simulink model "simulazione_sistema_lineare"  (R2025b)
settings: Solver=VariableStepAuto  StartTime=0.0  StopTime=10.0  RelTol=1e-3
values from neighbouring files (symbols this model uses):
  D_A = 1.5    [simulazione_sistema_non_lineare_code.m]
  D_F = zeros(1,4)    [simulazione_sistema_lineare_code.m]    (also in simulazione_sistema_non_lineare_code.m)
  G = tf(modello)    [tank_in_cascata_costanti.m]
  N_A = 0.1    [simulazione_sistema_non_lineare_code.m]
  N_F = zeros(1,4)    [simulazione_sistema_lineare_code.m]    (also in simulazione_sistema_non_lineare_code.m)
  RR = RR_s*RR_d    [tank_in_cascata_costanti.m]
  W = 3.5    [animazione_regolatore.m]    (also in simulazione_sistema_lineare_code.m = 1; simulazione_sistema_non_lineare_code.m = 1; tank_test_disturbo_dominio_complesso.m; tank_test_disturbo_dominio_tempo.m)
  x0 = [0,0]    [tank_animazione.m]
settings Model: Creator=lucia  LastModifiedBy=ecanf

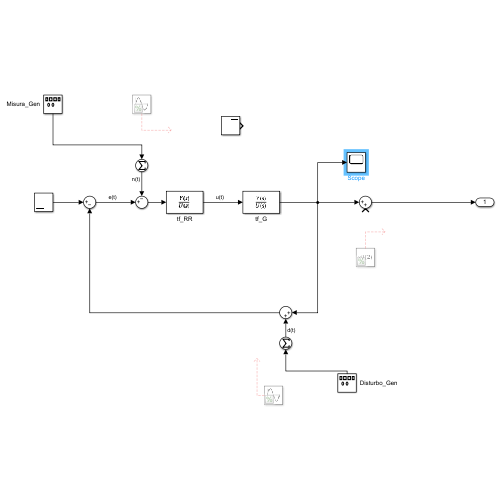
[thumbnail: Simulink's stored preview of the top-level diagram]
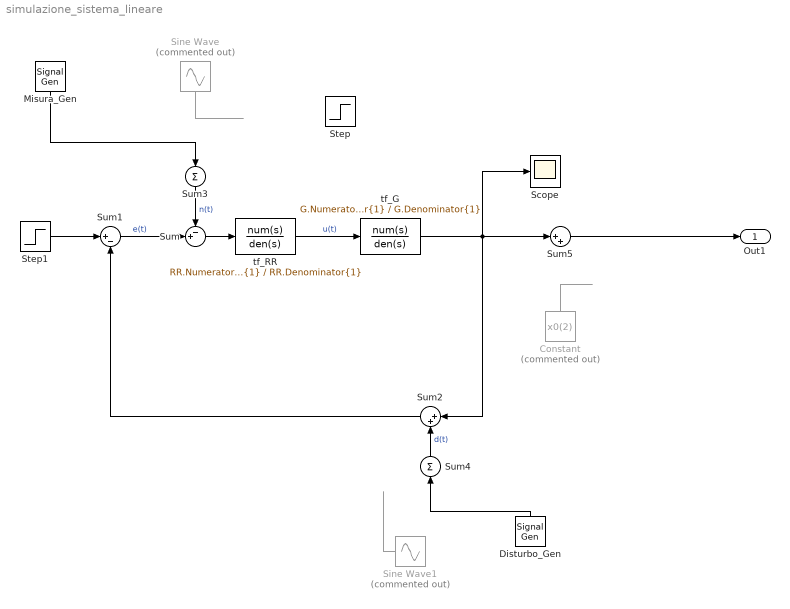
== system simulazione_sistema_lineare ==
  Constant : Constant  Commented=on  Value=x0(2)
  Disturbo_Gen : SignalGenerator  Amplitude="[1.5         1.5         1.5         1.5]"  Frequency="[0.4         0.8         1.2         1.6]"  Units=rad/sec
  Misura_Gen : SignalGenerator  Amplitude="[0.1         0.1         0.1         0.1]"  Frequency="[200000  400000  600000  800000]"  Units=rad/sec
  Scope : Scope
      settings: ActiveDisplayYMinimum=-3.4187225716841532  ActiveDisplayYMaximum=3.4108248657964362
  Sine Wave : Sin  Commented=on  Amplitude=N_A  Frequency=N_F  SampleTime=0
  Sine Wave1 : Sin  Commented=on  Amplitude=D_A  Frequency=D_F  SampleTime=0
  Step : Step  SampleTime=0
  Step1 : Step  Time=0  After=W  SampleTime=0
  Sum : Sum  Inputs=-+|
  Sum1 : Sum  Inputs=|+-
  Sum2 : Sum  Inputs=|++
  Sum3 : Sum  Inputs=+
  Sum4 : Sum  Inputs=+
  Sum5 : Sum  Inputs=|++
  tf_G : TransferFcn  Numerator=G.Numerator{1}  Denominator=G.Denominator{1}
  tf_RR : TransferFcn  Numerator=RR.Numerator{1}  Denominator=RR.Denominator{1}
  Out1 : Outport
  wires:
  tf_RR/1 -> tf_G/1  "u(t)"
  tf_G/1 -> Sum5/1, Scope/1, Sum2/1
  Sum1/1 -> Sum/2  "e(t)"
  Sum/1 -> tf_RR/1
  Misura_Gen/1 -> Sum3/1
  Disturbo_Gen/1 -> Sum4/1
  Sum2/1 -> Sum1/2
  Step1/1 -> Sum1/1
  Constant/1 -> ?
  Sum5/1 -> Out1/1
  Sine Wave/1 -> ?
  Sine Wave1/1 -> ?
  Sum3/1 -> Sum/1  "n(t)"
  Sum4/1 -> Sum2/2  "d(t)"
